simulink model "analise_de_estabilidade"  (R2023a)
settings: Solver=VariableStepAuto  StartTime=0.0  StopTime=25  RelTol=1e-3
settings Model: Creator=stem  LastModifiedBy=stem

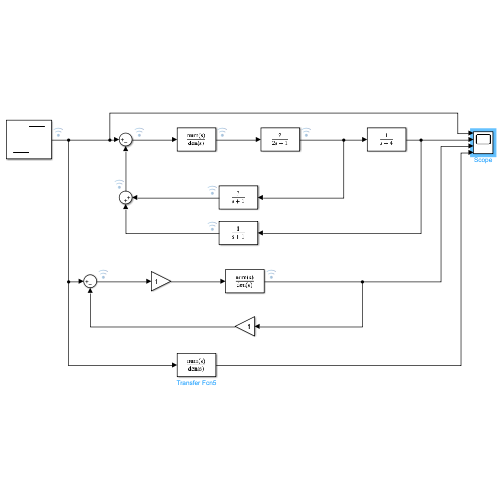
[thumbnail: Simulink's stored preview of the top-level diagram]
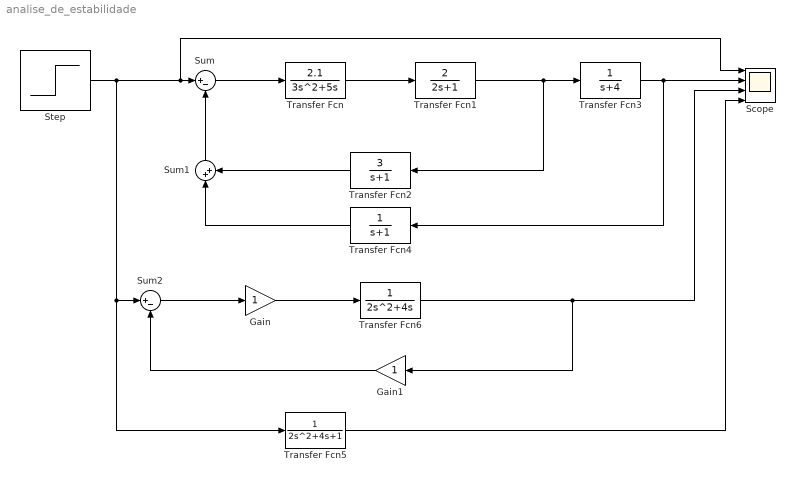
== system analise_de_estabilidade ==
  Gain : Gain
  Gain1 : Gain
  Scope : Scope  NumInputPorts=4
  Step : Step  Time=2  SampleTime=0
  Sum : Sum  Inputs=|+-
  Sum1 : Sum  Inputs=|++
  Sum2 : Sum  Inputs=|+-
  Transfer Fcn : TransferFcn  Numerator=2.1  Denominator=[3 5 0]
  Transfer Fcn1 : TransferFcn  Numerator=[2]  Denominator=[2 1]
  Transfer Fcn2 : TransferFcn  Numerator=[3]  Denominator=[1 1]
  Transfer Fcn3 : TransferFcn  Denominator=[1 4]
  Transfer Fcn4 : TransferFcn  Denominator=[1 1]
  Transfer Fcn5 : TransferFcn  Denominator=[2 4 1]
  Transfer Fcn6 : TransferFcn  Numerator=1  Denominator=[2 4 0]
  wires:
  Sum/1 -> Transfer Fcn/1
  Transfer Fcn/1 -> Transfer Fcn1/1
  Transfer Fcn1/1 -> Transfer Fcn2/1, Transfer Fcn3/1
  Transfer Fcn3/1 -> Transfer Fcn4/1, Scope/2
  Transfer Fcn6/1 -> Scope/3, Gain1/1
  Gain/1 -> Transfer Fcn6/1
  Step/1 -> Scope/1, Sum/1, Transfer Fcn5/1, Sum2/1
  Sum2/1 -> Gain/1
  Gain1/1 -> Sum2/2
  Sum1/1 -> Sum/2
  Transfer Fcn2/1 -> Sum1/2
  Transfer Fcn4/1 -> Sum1/1
  Transfer Fcn5/1 -> Scope/4
